simulink model "test_lift_motion_law"  (R2021b)
settings: Solver=VariableStepAuto  StartTime=0.0  StopTime=60  RelTol=1e-3
values from neighbouring files (symbols this model uses):
  CruiseVel = 2    [test_motion_law.m]
  MaxAcc = 2    [test_motion_law.m]
  MaxJerk = 8    [test_motion_law.m]
  switch_distance = 1    [test_motion_law.m]
  Ts = 1e-3    (= 0.001)    [test_motion_law.m]
libraries: simulink x1
settings Model: Creator=manue  LastModifiedBy=manue
settings ConfigComp: PLC_TargetIDE=generic  PLC_MultiTBSigbuilderTimeRange=off  PLC_InlineEnumCastFunction=off

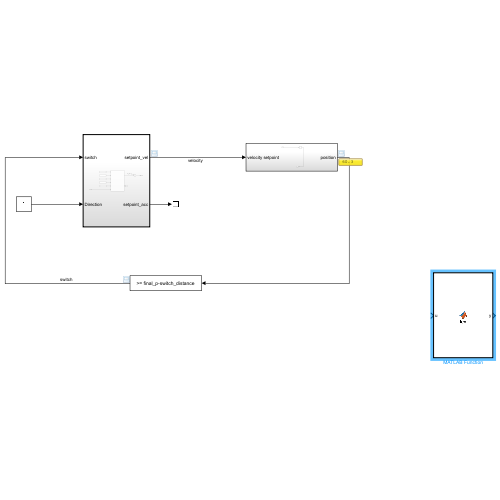
[thumbnail: Simulink's stored preview of the top-level diagram]
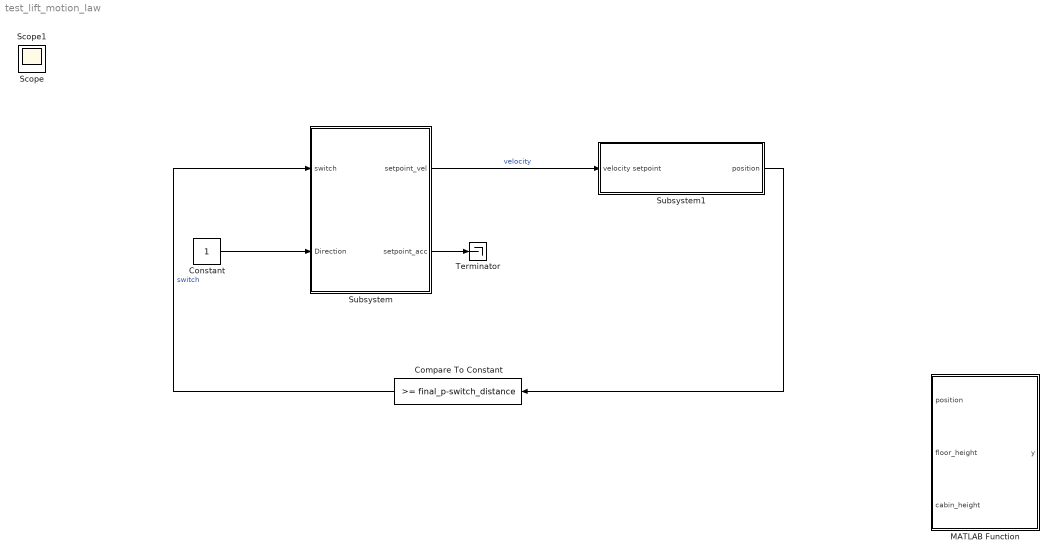
== system test_lift_motion_law ==
  Compare To Constant : simulink/Logic and Bit Operations/Compare To Constant  relop=>=  const=final_p-switch_distance  OutDataTypeStr=boolean
  Constant : Constant
  MATLAB Function : MATLAB Function  TreatAsAtomicUnit=on
  Subsystem : Subsystem  TreatAsAtomicUnit=on  SystemSampleTime=Ts
  Subsystem1 : Subsystem
  Terminator : Terminator
  Scope : Scope
  Scope1 : Scope
  wires:
  Compare To Constant/1 -> Subsystem/1(switch)  "switch"
  Constant/1 -> Subsystem/2(Direction)
  Subsystem/2(setpoint_acc) -> Terminator/1
  Subsystem1/1(position) -> Compare To Constant/1
  Subsystem/1(setpoint_vel) -> Subsystem1/1(velocity setpoint)  "velocity"

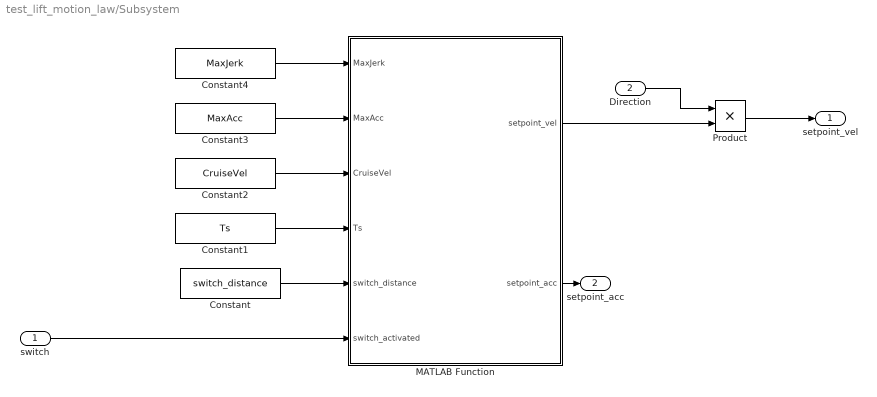
== system test_lift_motion_law/Subsystem ==
  switch : Inport
  Direction : Inport  Port=2
  Constant : Constant  Value=switch_distance
  Constant1 : Constant  Value=Ts
  Constant2 : Constant  Value=CruiseVel
  Constant3 : Constant  Value=MaxAcc
  Constant4 : Constant  Value=MaxJerk
  MATLAB Function : MATLAB Function  TreatAsAtomicUnit=on
  Product : Product
  setpoint_vel : Outport
  setpoint_acc : Outport  Port=2
  wires:
  Constant2/1 -> MATLAB Function/3(CruiseVel)
  Constant/1 -> MATLAB Function/5(switch_distance)
  Constant1/1 -> MATLAB Function/4(Ts)
  switch/1 -> MATLAB Function/6(switch_activated)
  Constant3/1 -> MATLAB Function/2(MaxAcc)
  Constant4/1 -> MATLAB Function/1(MaxJerk)
  MATLAB Function/2(setpoint_acc) -> setpoint_acc/1
  MATLAB Function/1(setpoint_vel) -> Product/2
  Product/1 -> setpoint_vel/1
  Direction/1 -> Product/1

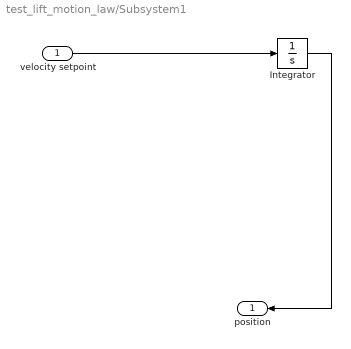
== system test_lift_motion_law/Subsystem1 ==
  velocity setpoint : Inport
  Integrator : Integrator
  position : Outport
  wires:
  Integrator/1 -> position/1
  velocity setpoint/1 -> Integrator/1

== matlab function test_lift_motion_law/MATLAB Function ==
  data: position input; y output; floor_height input; cabin_height input
function y = SwitchSensors(position,floor_height,cabin_height)

== matlab function test_lift_motion_law/Subsystem/MATLAB Function ==
  data: MaxJerk input; setpoint_vel output; MaxAcc input; CruiseVel input; Ts input; switch_distance input; switch_activated input; setpoint_acc output
function [setpoint_vel, setpoint_acc] = MotionLaw(MaxJerk, MaxAcc, CruiseVel, Ts, switch_distance, switch_activated)

persistent state vel acc pos
if isempty(state)
    state=1;
    vel=0;
    acc=0;
    pos=0;
end

% compute deceleration distance: 
% case 1: the maximum acceleration is reached
% case 2: the maximum acceleration is not reached
if (CruiseVel^(1/2)*MaxJerk^(1/2)>MaxAcc) % case 1
    deceleration_distance=(CruiseVel*(MaxAcc^2 + CruiseVel*MaxJerk))/(2*MaxAcc*MaxJerk);
else % case 2
    deceleration_distance =CruiseVel^(3/2)/MaxJerk^(1/2);
end

if (state==1)  %increase acceleration
    jerk=MaxJerk;
elseif (state==2) % max acceleration
    jerk=0;
elseif (state==3) % decrease acceleration
    jerk=-MaxJerk;
elseif (state==4) % keep cruise velocity
    jerk=0;
elseif (state==5) % kep cruise velocity, switch has been triggered
    jerk=0;
elseif (state==6) % decrease acceleration (to slow down speed)
    jerk=-MaxJerk;
elseif (state==7) % max negative acceleration (to slow down speed)
    jerk=0;
elseif (state==8) % increase acceleration (to return to null acceleration)
    jerk=MaxJerk;
else % steaty-state case
    jerk=0;
    vel=0;
    acc=0;
end


pos=pos+vel*Ts+0.5*acc*Ts^2+1.0/6.0*jerk*Ts^3; % traveled distance
vel=vel+acc*Ts+0.5*Ts*Ts*jerk; % velocity
acc=acc+Ts*jerk; % acceleration

limit_velocity=CruiseVel-acc^2/(2*MaxJerk); % velocity limit to start removing accelaration to reach cruise velocity
limit_velocity_final=acc^2/(2*MaxJerk); % velocity limit to start removing accelaration to reach null velocity

%% state machine transition 
if (state==1 && acc>=MaxAcc) % max acceleration reached
    state=2;
    acc=min(acc,MaxAcc);
elseif ((state==2 || state==1) && vel>=limit_velocity) % limit velocity reached
    state=3;
elseif (state==3 && acc<=0) % null acceleration reached
    state=4;
    acc=0;
elseif (state==4 && switch_activated) % switch has been triggered
    state=5;
    pos=0;
elseif (state==5 && pos>=(switch_distance-deceleration_distance)) % time to slow down
    state=6;
elseif (state==6 && acc<=-MaxAcc) % negative max acceleration reached
    state=7;
    acc=max(acc,-MaxAcc);
elseif ((state==7 || state==6) && vel<=limit_velocity_final) % limit acceleration to stop motion is reached
    state=8;
elseif (state==8 && vel<=0) % steady state reached
    state=0;
    vel=0;
    acc=0;
end


setpoint_vel=vel;
setpoint_acc=acc;
